simulink model "Mdl_Tacho"  (R2024b)
settings: Solver=FixedStepDiscrete  StartTime=0.0  StopTime=10.0  FixedStep=0.1  RelTol=1e-3  EnableMultiTasking=on
values from neighbouring files (symbols this model uses):
  EQUIPPED_FLAG = mpt.Parameter    [Mdl_Tacho_DD.m]
  HV_NE = mpt.Parameter    [Mdl_Tacho_DD.m]
  MCUID0025 = mpt.Parameter    [Mdl_Tacho_DD.m]
  MCUID0025_MAX = mpt.Parameter    [Mdl_Tacho_DD.m]
  MCUID0639 = mpt.Parameter    [Mdl_Tacho_DD.m]
  MCUID0640 = mpt.Parameter    [Mdl_Tacho_DD.m]
  Mdl_Tacho_cTaskPeriod = mpt.Parameter    [Mdl_Tacho_rte_types.m]
  N1 = mpt.Parameter    [Mdl_Tacho_DD.m]
  N2 = mpt.Parameter    [Mdl_Tacho_DD.m]
  NE1 = mpt.Parameter    [Mdl_Tacho_DD.m]
  NE_MET = mpt.Parameter    [Mdl_Tacho_DD.m]
  NE_MET_INVALID = mpt.Parameter    [Mdl_Tacho_DD.m]
  PTSYS_48V = mpt.Parameter    [Mdl_Tacho_DD.m]
  PTSYS_CONV = mpt.Parameter    [Mdl_Tacho_DD.m]
  PTSYS_DEFAULT = mpt.Parameter    [Mdl_Tacho_DD.m]
  PTSYS_HV = mpt.Parameter    [Mdl_Tacho_DD.m]
  PTSYS_MOTORHV = mpt.Parameter    [Mdl_Tacho_DD.m]
  PTSYS_PHV = mpt.Parameter    [Mdl_Tacho_DD.m]
  PTSYS_S_S = mpt.Parameter    [Mdl_Tacho_DD.m]
  REDZONE_MAX_VAL = mpt.Parameter    [Mdl_Tacho_DD.m]
  REDZONE_MIN_VAL = mpt.Parameter    [Mdl_Tacho_DD.m]
  RTE_E_MAX_AGE_EXCEEDED = mpt.Parameter    [Mdl_Tacho_rte_types.m]
  RTE_E_NEVER_RECEIVED = mpt.Parameter    [Mdl_Tacho_rte_types.m]
  RTE_E_OK = mpt.Parameter    [Mdl_Tacho_rte_types.m]
  RZ_INIT_VAL = mpt.Parameter    [Mdl_Tacho_DD.m]
  SPD_THRESHOLD = mpt.Parameter    [Mdl_Tacho_DD.m]
  TACHO_070D = mpt.Parameter    [Mdl_Tacho_DD.m]
  TACHO_COUNT_INIT = mpt.Parameter    [Mdl_Tacho_DD.m]
  TACHO_COUNT_INIT_U16 = mpt.Parameter    [Mdl_Tacho_DD.m]
  TACHO_COUNT_ONE = mpt.Parameter    [Mdl_Tacho_DD.m]
  TACHO_COUNT_TWO = mpt.Parameter    [Mdl_Tacho_DD.m]
  TACHO_DEBOUNCE_TIME = mpt.Parameter    [Mdl_Tacho_DD.m]
  TACHO_DISABLE = mpt.Parameter    [Mdl_Tacho_DD.m]
  TACHO_ENABLE = mpt.Parameter    [Mdl_Tacho_DD.m]
  TACHO_F = mpt.Parameter    [Mdl_Tacho_DD.m]
  TACHO_FSPORT = mpt.Parameter    [Mdl_Tacho_DD.m]
  TACHO_GR = mpt.Parameter    [Mdl_Tacho_DD.m]
  TACHO_GRMN = mpt.Parameter    [Mdl_Tacho_DD.m]
  TACHO_HYS_MAX = mpt.Parameter    [Mdl_Tacho_DD.m]
  TACHO_HYS_MIN = mpt.Parameter    [Mdl_Tacho_DD.m]
  TACHO_OFF = mpt.Parameter    [Mdl_Tacho_DD.m]
  TACHO_ON = mpt.Parameter    [Mdl_Tacho_DD.m]
  TACHO_RES_DIVIDER = mpt.Parameter    [Mdl_Tacho_DD.m]
  TACHO_RESOLUTION = mpt.Parameter    [Mdl_Tacho_DD.m]
  TACHO_REV_PEAK_TIMER_ELAPSED = mpt.Parameter    [Mdl_Tacho_DD.m]
  TACHO_RPM_THRESHOLD = mpt.Parameter    [Mdl_Tacho_DD.m]
  TACHO_TEN = mpt.Parameter    [Mdl_Tacho_DD.m]
  TACHO_THRESHOLD = mpt.Parameter    [Mdl_Tacho_DD.m]
  TACHO_VAL_ONE = mpt.Parameter    [Mdl_Tacho_DD.m]
  TACHO_VAL_ONE_U16 = mpt.Parameter    [Mdl_Tacho_DD.m]
  TACHO_VAL_TEN = mpt.Parameter    [Mdl_Tacho_DD.m]
  TACHO_VAL_THREE = mpt.Parameter    [Mdl_Tacho_DD.m]
  TACHO_VAL_TWENTY = mpt.Parameter    [Mdl_Tacho_DD.m]
  TACHO_VAL_ZERO = mpt.Parameter    [Mdl_Tacho_DD.m]
  TACHO_VAL_ZERO_U16 = mpt.Parameter    [Mdl_Tacho_DD.m]
  TACHO_VAL_ZERO_U32 = mpt.Parameter    [Mdl_Tacho_DD.m]
  VAL_ONE = mpt.Parameter    [Mdl_Tacho_DD.m]
  VAL_ZERO = mpt.Parameter    [Mdl_Tacho_DD.m]
undefined symbols (not defined in the file or in its folder): CLUSTER_ACTIVE, CLUSTER_INACTIVE, eEngineSpeedIn, eFUNC_NORTH_AMERICA, eJust_Received, eSIGNAL_MISSING, eSIGNAL_NEVER_RECEIVED, IgnOff, IgnOn, NE1_Recieve_Notify_Value, NE1_SignalVal, pJustRcvdStatus, RxCan_SignalClearJustRcvdStatus, RxCan_SignalGetJustRcvdStatus, RxCan_SignalInvalidProcessingControl, RxCan_SignalMissingProcessingControl, RxCan_SignalNRProcessingControl, SignalId, Status, tRxSignalId_type_instance, tRxSignalJustRcvdStatus_type_instance, tRxSignalStatus_type_instance
libraries: simulink x23
(part 2 of 3)

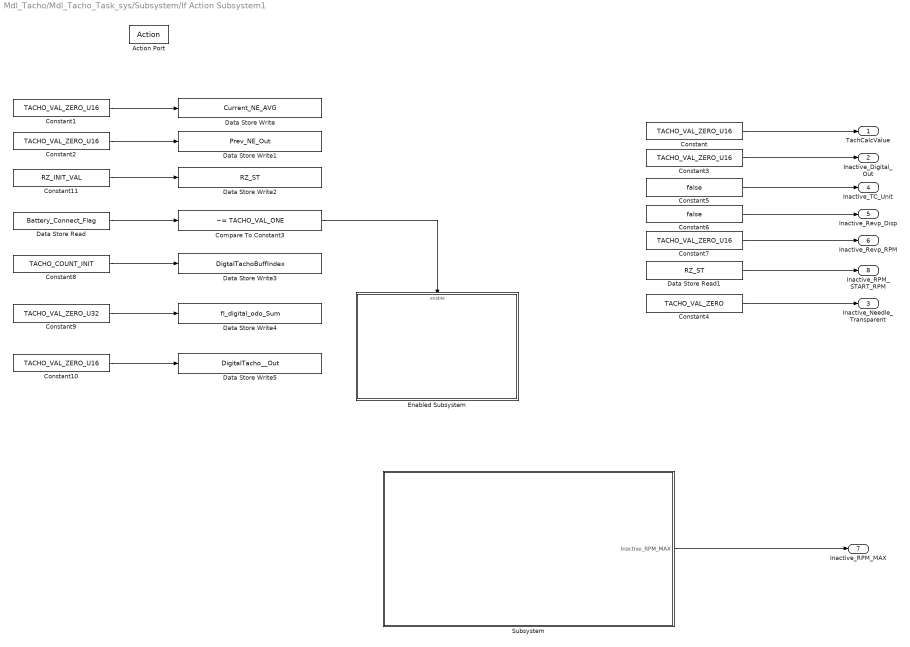
== system Mdl_Tacho/Mdl_Tacho_Task_sys/Subsystem/If Action Subsystem1 ==
  Action Port : ActionPort  ActionPortLabel=else
  Compare To Constant3 : simulink/Logic and Bit Operations/Compare To Constant  relop=~=  const=TACHO_VAL_ONE  OutDataTypeStr=boolean
  Constant{,1..3} (4 alike) : Constant  Value=TACHO_VAL_ZERO_U16  OutDataTypeStr=uint16  LockScale=on
  Constant10 : Constant  Value=TACHO_VAL_ZERO_U16  LockScale=on
  Constant11 : Constant  Value=RZ_INIT_VAL
  Constant4 : Constant  Value=TACHO_VAL_ZERO  LockScale=on
  Constant5 : Constant  Value=false  LockScale=on
  Constant6 : Constant  Value=false  LockScale=on
  Constant7 : Constant  Value=TACHO_VAL_ZERO_U16  LockScale=on
  Constant8 : Constant  Value=TACHO_COUNT_INIT
  Constant9 : Constant  Value=TACHO_VAL_ZERO_U32  LockScale=on
  Data Store Read : DataStoreRead  DataStoreName=Battery_Connect_Flag  IndexOptions=Index vector (dialog)  Indices=1  OutputSizes=1
  Data Store Read1 : DataStoreRead  DataStoreName=RZ_ST  IndexOptions=Index vector (dialog)  Indices=1  OutputSizes=1
  Data Store Write : DataStoreWrite  DataStoreName=Current_NE_AVG  IndexOptions=Index vector (dialog)  Indices=1  OutputSizes=1
  Data Store Write1 : DataStoreWrite  DataStoreName=Prev_NE_Out  IndexOptions=Index vector (dialog)  Indices=1  OutputSizes=1
  Data Store Write2 : DataStoreWrite  DataStoreName=RZ_ST  IndexOptions=Index vector (dialog)  Indices=1  OutputSizes=1
  Data Store Write3 : DataStoreWrite  DataStoreName=DigtalTachoBuffIndex  IndexOptions=Index vector (dialog)  Indices=1  OutputSizes=1
  Data Store Write4 : DataStoreWrite  DataStoreName=fl_digital_odo_Sum  IndexOptions=Index vector (dialog)  Indices=1  OutputSizes=1
  Data Store Write5 : DataStoreWrite  DataStoreName=DigitalTacho__Out  IndexOptions=Index vector (dialog)  Indices=1  OutputSizes=1
  Enabled Subsystem : Subsystem  Priority=0  TreatAsAtomicUnit=on
  Subsystem : Subsystem  Priority=1
  TachCalcValue : Outport  VectorParamsAs1DForOutWhenUnconnected=off
  Inactive_Digital_Out : Outport  Port=2  VectorParamsAs1DForOutWhenUnconnected=off
  Inactive_Needle_Transparent : Outport  Port=3  VectorParamsAs1DForOutWhenUnconnected=off
  Inactive_TC_Unit : Outport  Port=4  VectorParamsAs1DForOutWhenUnconnected=off
  Inactive_Revp_Disp : Outport  Port=5  VectorParamsAs1DForOutWhenUnconnected=off
  Inactive_Revp_RPM : Outport  Port=6  VectorParamsAs1DForOutWhenUnconnected=off
  Inactive_RPM_MAX : Outport  Port=7  VectorParamsAs1DForOutWhenUnconnected=off
  Inactive_RPM_START_RPM : Outport  Port=8  VectorParamsAs1DForOutWhenUnconnected=off
  wires:
  Constant/1 -> TachCalcValue/1
  Constant1/1 -> Data Store Write/1
  Constant2/1 -> Data Store Write1/1
  Constant3/1 -> Inactive_Digital_Out/1
  Constant4/1 -> Inactive_Needle_Transparent/1
  Constant5/1 -> Inactive_TC_Unit/1
  Constant6/1 -> Inactive_Revp_Disp/1
  Constant7/1 -> Inactive_Revp_RPM/1
  Data Store Read1/1 -> Inactive_RPM_START_RPM/1
  Constant11/1 -> Data Store Write2/1
  Data Store Read/1 -> Compare To Constant3/1
  Compare To Constant3/1 -> Enabled Subsystem/Enable
  Constant8/1 -> Data Store Write3/1
  Constant9/1 -> Data Store Write4/1
  Constant10/1 -> Data Store Write5/1
  Subsystem/1(Inactive_RPM_MAX) -> Inactive_RPM_MAX/1

== system Mdl_Tacho/Mdl_Tacho_Task_sys/Subsystem/NE1_Missing_Notify ==
  NE1_COMStatus : Inport
  NE1_Value : Inport  Port=2
  NE1_In_JR : Inport  Port=3
  Compare To Constant1 : simulink/Logic and Bit Operations/Compare To Constant  relop=~=  const=RTE_E_MAX_AGE_EXCEEDED  OutDataTypeStr=boolean
  If : If  IfExpression=u1 ~= 0
  If Action Subsystem : Subsystem  TreatAsAtomicUnit=on
  If Action Subsystem1 : Subsystem  TreatAsAtomicUnit=on
  Merge : Merge
  NE1_Status : Outport  VectorParamsAs1DForOutWhenUnconnected=off
  wires:
  NE1_COMStatus/1 -> Compare To Constant1/1
  Compare To Constant1/1 -> If/1
  If/1 -> If Action Subsystem/Action
  NE1_In_JR/1 -> If Action Subsystem/1(NE1_In_JR)
  If Action Subsystem/1(NE1_Status) -> Merge/1
  If Action Subsystem1/1(NE1_Status) -> Merge/2
  Merge/1 -> NE1_Status/1
  If/2 -> If Action Subsystem1/Action
  NE1_Value/1 -> If Action Subsystem/2(NE1_Value)

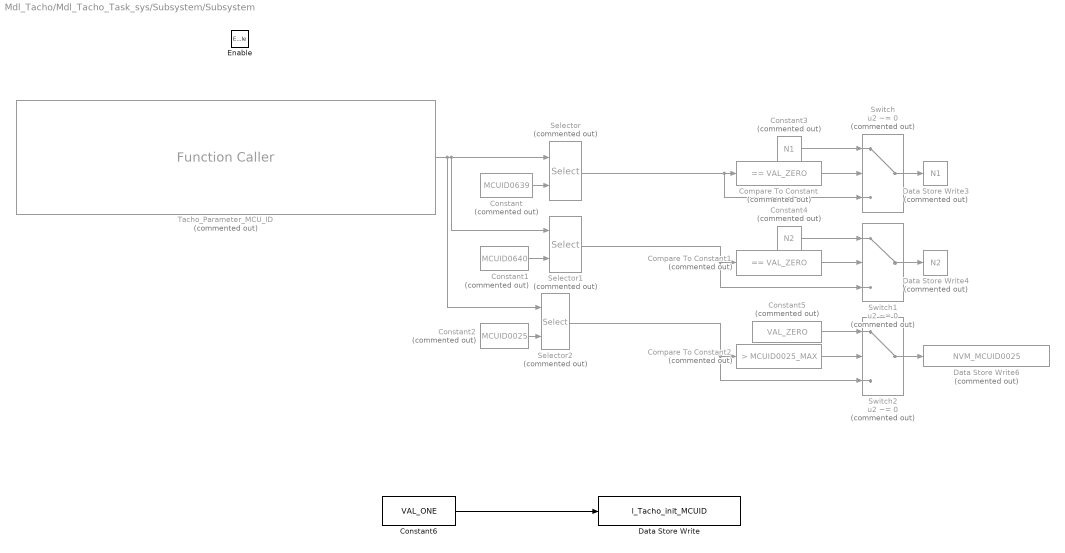
== system Mdl_Tacho/Mdl_Tacho_Task_sys/Subsystem/Subsystem ==
  Enable : EnablePort
  Compare To Constant : simulink/Logic and Bit Operations/Compare To Constant  Commented=on  relop===  const=VAL_ZERO  OutDataTypeStr=boolean
  Compare To Constant1 : simulink/Logic and Bit Operations/Compare To Constant  Commented=on  relop===  const=VAL_ZERO  OutDataTypeStr=boolean
  Compare To Constant2 : simulink/Logic and Bit Operations/Compare To Constant  Commented=on  relop=>  const=MCUID0025_MAX  OutDataTypeStr=boolean
  Constant : Constant  Commented=on  Value=MCUID0639
  Constant1 : Constant  Commented=on  Value=MCUID0640
  Constant2 : Constant  Commented=on  Value=MCUID0025
  Constant3 : Constant  Commented=on  Value=N1
  Constant4 : Constant  Commented=on  Value=N2
  Constant5 : Constant  Commented=on  Value=VAL_ZERO
  Constant6 : Constant  Value=VAL_ONE
  Data Store Write : DataStoreWrite  DataStoreName=l_Tacho_init_MCUID  IndexOptions=Index vector (dialog)  Indices=1  OutputSizes=1
  Data Store Write3 : DataStoreWrite  Commented=on  DataStoreName=N1  IndexOptions=Index vector (dialog)  Indices=1  OutputSizes=1
  Data Store Write4 : DataStoreWrite  Commented=on  DataStoreName=N2  IndexOptions=Index vector (dialog)  Indices=1  OutputSizes=1
  Data Store Write6 : DataStoreWrite  Commented=on  DataStoreName=NVM_MCUID0025  IndexOptions=Index vector (dialog)  Indices=1  OutputSizes=1
  Selector : Selector  Commented=on  IndexMode=Zero-based  InputPortWidth=6  IndexOptions=Index vector (port)  Indices=[1 3]  OutputSizes=1
  Selector1 : Selector  Commented=on  IndexMode=Zero-based  InputPortWidth=6  IndexOptions=Index vector (port)  Indices=[1 3]  OutputSizes=1
  Selector2 : Selector  Commented=on  IndexMode=Zero-based  InputPortWidth=6  IndexOptions=Index vector (port)  Indices=[1 3]  OutputSizes=1
  Switch : Switch  Commented=on  Criteria=u2 ~= 0  OutDataTypeStr=uint16  SaturateOnIntegerOverflow=off  InputSameDT=off
  Switch1 : Switch  Commented=on  Criteria=u2 ~= 0  OutDataTypeStr=uint16  SaturateOnIntegerOverflow=off  InputSameDT=off
  Switch2 : Switch  Commented=on  Criteria=u2 ~= 0  OutDataTypeStr=uint8  SaturateOnIntegerOverflow=off  InputSameDT=off
  Tacho_Parameter_MCU_ID : FunctionCaller  Commented=on  FunctionPrototype=pMCUCONST_Data = Tacho_Parameter_MCU_ID()  InputArgumentSpecifications=<Enter example>  OutputArgumentSpecifications=uint16(zeros(1,6))
  wires:
  Constant/1 -> Selector/2
  Constant1/1 -> Selector1/2
  Constant2/1 -> Selector2/2
  Selector/1 -> Switch/3, Compare To Constant/1
  Compare To Constant/1 -> Switch/2
  Compare To Constant1/1 -> Switch1/2
  Constant3/1 -> Switch/1
  Switch/1 -> Data Store Write3/1
  Constant4/1 -> Switch1/1
  Selector1/1 -> Switch1/3, Compare To Constant1/1
  Switch1/1 -> Data Store Write4/1
  Constant5/1 -> Switch2/1
  Compare To Constant2/1 -> Switch2/2
  Selector2/1 -> Switch2/3, Compare To Constant2/1
  Switch2/1 -> Data Store Write6/1
  Tacho_Parameter_MCU_ID/1 -> Selector1/1, Selector/1, Selector2/1
  Constant6/1 -> Data Store Write/1

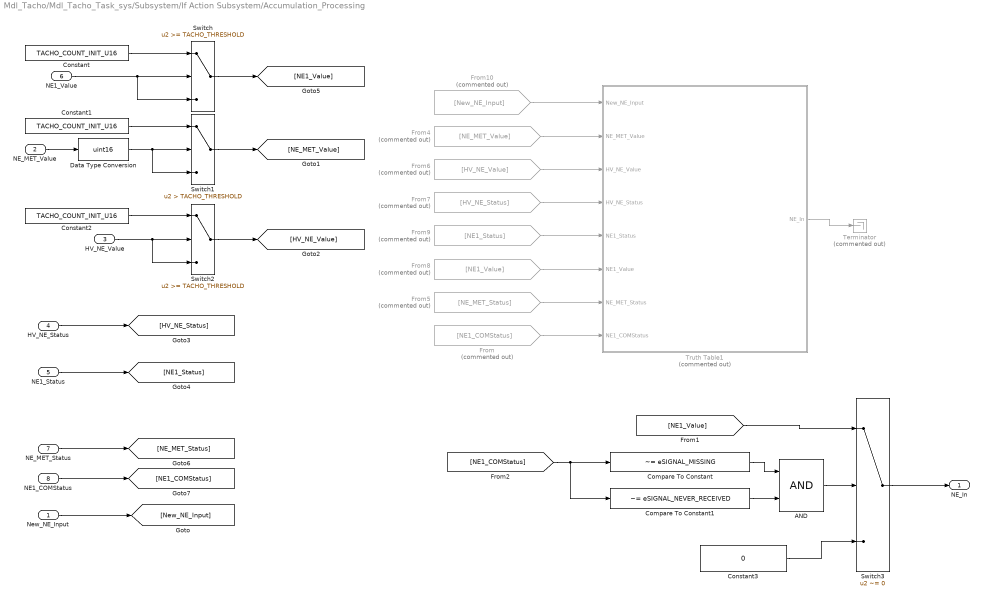
== system Mdl_Tacho/Mdl_Tacho_Task_sys/Subsystem/If Action Subsystem/Accumulation_Processing ==
  New_NE_Input : Inport
  NE_MET_Value : Inport  Port=2
  HV_NE_Value : Inport  Port=3
  HV_NE_Status : Inport  Port=4
  NE1_Status : Inport  Port=5
  NE1_Value : Inport  Port=6
  NE_MET_Status : Inport  Port=7
  NE1_COMStatus : Inport  Port=8
  AND : Logic  AllPortsSameDT=off  OutDataTypeStr=boolean
  Compare To Constant : simulink/Logic and Bit Operations/Compare To Constant  relop=~=  const=eSIGNAL_MISSING  OutDataTypeStr=boolean
  Compare To Constant1 : simulink/Logic and Bit Operations/Compare To Constant  relop=~=  const=eSIGNAL_NEVER_RECEIVED  OutDataTypeStr=boolean
  Constant : Constant  Value=TACHO_COUNT_INIT_U16
  Constant1 : Constant  Value=TACHO_COUNT_INIT_U16
  Constant2 : Constant  Value=TACHO_COUNT_INIT_U16
  Constant3 : Constant  Value=0
  Data Type Conversion : DataTypeConversion  OutDataTypeStr=uint16  SaturateOnIntegerOverflow=off  RndMeth=Floor
  From : From  Commented=on  GotoTag=NE1_COMStatus
  From10 : From  Commented=on  GotoTag=New_NE_Input
  From4 : From  Commented=on  GotoTag=NE_MET_Value
  From5 : From  Commented=on  GotoTag=NE_MET_Status
  From6 : From  Commented=on  GotoTag=HV_NE_Value
  From7 : From  Commented=on  GotoTag=HV_NE_Status
  From8 : From  Commented=on  GotoTag=NE1_Value
  From9 : From  Commented=on  GotoTag=NE1_Status
  Switch : Switch  Threshold=TACHO_THRESHOLD  OutDataTypeStr=uint16  SaturateOnIntegerOverflow=off  InputSameDT=off
  Switch1 : Switch  Criteria=u2 > Threshold  Threshold=TACHO_THRESHOLD  SaturateOnIntegerOverflow=off  InputSameDT=off
  Switch2 : Switch  Threshold=TACHO_THRESHOLD  SaturateOnIntegerOverflow=off  InputSameDT=off
  Switch3 : Switch  Criteria=u2 ~= 0  OutDataTypeStr=uint16  SaturateOnIntegerOverflow=off  InputSameDT=off
  Terminator : Terminator  Commented=on
  Truth Table1 : Truth Table  Commented=on  TreatAsAtomicUnit=on
  NE_In : Outport  VectorParamsAs1DForOutWhenUnconnected=off
  wires:
  From6/1 -> Truth Table1/3(HV_NE_Value)
  From9/1 -> Truth Table1/5(NE1_Status)
  From5/1 -> Truth Table1/7(NE_MET_Status)
  From7/1 -> Truth Table1/4(HV_NE_Status)
  From10/1 -> Truth Table1/1(New_NE_Input)
  From4/1 -> Truth Table1/2(NE_MET_Value)
  From8/1 -> Truth Table1/6(NE1_Value)
  HV_NE_Status/1 -> [HV_NE_Status]
  NE1_Status/1 -> [NE1_Status]
  NE_MET_Status/1 -> [NE_MET_Status]
  NE1_COMStatus/1 -> [NE1_COMStatus]
  From/1 -> Truth Table1/8(NE1_COMStatus)
  Constant/1 -> Switch/1
  Switch1/1 -> [NE_MET_Value]
  Constant1/1 -> Switch1/1
  NE_MET_Value/1 -> Data Type Conversion/1
  HV_NE_Value/1 -> Switch2/3, Switch2/2
  Constant2/1 -> Switch2/1
  Switch2/1 -> [HV_NE_Value]
  New_NE_Input/1 -> [New_NE_Input]
  Switch/1 -> [NE1_Value]
  NE1_Value/1 -> Switch/3, Switch/2
  [NE1_COMStatus] -> Compare To Constant1/1, Compare To Constant/1
  Compare To Constant/1 -> AND/1
  Compare To Constant1/1 -> AND/2
  Switch3/1 -> NE_In/1
  AND/1 -> Switch3/2
  [NE1_Value] -> Switch3/1
  Constant3/1 -> Switch3/3
  Truth Table1/1(NE_In) -> Terminator/1
  Data Type Conversion/1 -> Switch1/3, Switch1/2

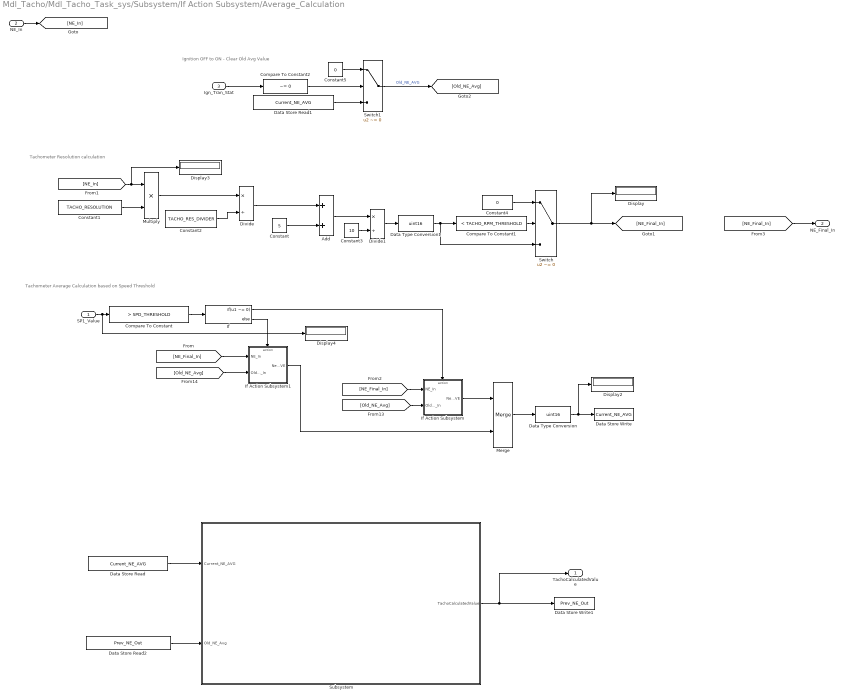
== system Mdl_Tacho/Mdl_Tacho_Task_sys/Subsystem/If Action Subsystem/Average_Calculation ==
  note: Tachometer Average Calculation based on Speed Threshold
  note: Tachometer Resolution calculation
  note: Ignition OFF to ON - Clear Old Avg Value
  SP1_Value : Inport
  NE_In : Inport  Port=2
  Ign_Tran_Stat : Inport  Port=3
  Add : Sum  OutDataTypeStr=uint32  RndMeth=Simplest
  Compare To Constant : simulink/Logic and Bit Operations/Compare To Constant  relop=>  const=SPD_THRESHOLD  OutDataTypeStr=boolean
  Compare To Constant1 : simulink/Logic and Bit Operations/Compare To Constant  relop=<  const=TACHO_RPM_THRESHOLD  OutDataTypeStr=boolean
  Compare To Constant2 : simulink/Logic and Bit Operations/Compare To Constant  relop=~=  const=0  OutDataTypeStr=boolean
  Constant : Constant  Value=5  OutDataTypeStr=uint16  LockScale=on
  Constant1 : Constant  Value=TACHO_RESOLUTION  OutDataTypeStr=uint32  LockScale=on
  Constant2 : Constant  Value=TACHO_RES_DIVIDER  OutDataTypeStr=uint32  LockScale=on
  Constant3 : Constant  Value=10  OutDataTypeStr=uint16  LockScale=on
  Constant4 : Constant  Value=0  OutDataTypeStr=uint16  LockScale=on
  Constant5 : Constant  Value=0  OutDataTypeStr=uint16
  Data Store Read : DataStoreRead  DataStoreName=Current_NE_AVG  IndexOptions=Index vector (dialog)  Indices=1  OutputSizes=1
  Data Store Read1 : DataStoreRead  DataStoreName=Current_NE_AVG  IndexOptions=Index vector (dialog)  Indices=1  OutputSizes=1
  Data Store Read2 : DataStoreRead  DataStoreName=Prev_NE_Out  IndexOptions=Index vector (dialog)  Indices=1  OutputSizes=1
  Data Store Write : DataStoreWrite  DataStoreName=Current_NE_AVG  IndexOptions=Index vector (dialog)  Indices=1  OutputSizes=1
  Data Store Write1 : DataStoreWrite  DataStoreName=Prev_NE_Out  IndexOptions=Index vector (dialog)  Indices=1  OutputSizes=1
  Data Type Conversion : DataTypeConversion  OutDataTypeStr=uint16  RndMeth=Simplest  SaturateOnIntegerOverflow=off
  Data Type Conversion1 : DataTypeConversion  OutDataTypeStr=uint16  RndMeth=Simplest  SaturateOnIntegerOverflow=off
  Display{,2..4} (4 alike) : Display
  Divide : Product  Inputs=*/  OutDataTypeStr=uint32  RndMeth=Simplest
  Divide1 : Product  Inputs=*/  OutDataTypeStr=uint32  RndMeth=Simplest
  If : If  Priority=3  IfExpression=u1 ~= 0
  If Action Subsystem : Subsystem  TreatAsAtomicUnit=on
  If Action Subsystem1 : Subsystem  TreatAsAtomicUnit=on
  Merge : Merge
  Multiply : Product  OutDataTypeStr=uint32  RndMeth=Simplest  LockScale=on
  Subsystem : Subsystem  Priority=4  TreatAsAtomicUnit=on  RTWFcnName=Mdl_Tacho_Hysteris_Process_Output
      settings: RTWSystemCode=Nonreusable function  RTWFcnNameOpts=User specified
  Switch : Switch  Priority=2  Criteria=u2 ~= 0  OutDataTypeStr=uint16  RndMeth=Simplest  SaturateOnIntegerOverflow=off  InputSameDT=off
  Switch1 : Switch  Priority=1  Criteria=u2 ~= 0  OutDataTypeStr=uint16  RndMeth=Simplest  SaturateOnIntegerOverflow=off  InputSameDT=off
  TachoCalculatedValue : Outport  VectorParamsAs1DForOutWhenUnconnected=off
  NE_Final_In : Outport  Port=2  VectorParamsAs1DForOutWhenUnconnected=off
  wires:
  If Action Subsystem/1(New NE_AVE) -> Merge/1
  [NE_Final_In] -> If Action Subsystem/1(NE_In)
  If/1 -> If Action Subsystem/Action
  [Old_NE_Avg] -> If Action Subsystem/2(Old_NE_In)
  If/2 -> If Action Subsystem1/Action
  Merge/1 -> Data Type Conversion/1
  Compare To Constant/1 -> If/1
  [Old_NE_Avg] -> If Action Subsystem1/2(Old_NE_In)
  If Action Subsystem1/1(New NE_AVE) -> Merge/2
  NE_In/1 -> [NE_In]
  Constant1/1 -> Multiply/2
  [NE_Final_In] -> If Action Subsystem1/1(NE_In)
  Multiply/1 -> Divide/1
  Constant2/1 -> Divide/2
  Divide/1 -> Add/1
  Constant/1 -> Add/2
  Add/1 -> Divide1/1
  Constant3/1 -> Divide1/2
  Divide1/1 -> Data Type Conversion1/1
  Compare To Constant1/1 -> Switch/2
  Constant4/1 -> Switch/1
  Switch/1 -> Display/1, [NE_Final_In]
  Ign_Tran_Stat/1 -> Compare To Constant2/1
  Compare To Constant2/1 -> Switch1/2
  Switch1/1 -> [Old_NE_Avg]  "Old_NE_AVG"
  Constant5/1 -> Switch1/1
  Data Store Read1/1 -> Switch1/3
  Data Type Conversion1/1 -> Compare To Constant1/1, Switch/3
  SP1_Value/1 -> Display4/1, Compare To Constant/1
  Data Store Read/1 -> Subsystem/1(Current_NE_AVG)
  Data Store Read2/1 -> Subsystem/2(Old_NE_Avg)
  Subsystem/1(TachoCalculatedValue) -> Data Store Write1/1, TachoCalculatedValue/1
  Data Type Conversion/1 -> Display2/1, Data Store Write/1
  [NE_In] -> Display3/1, Multiply/1
  [NE_Final_In] -> NE_Final_In/1

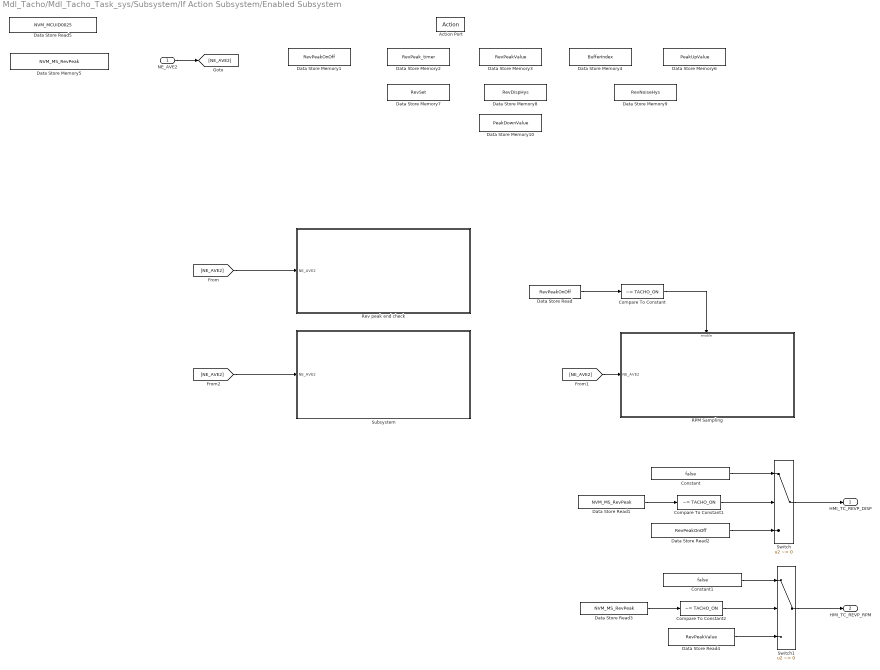
== system Mdl_Tacho/Mdl_Tacho_Task_sys/Subsystem/If Action Subsystem/Enabled Subsystem ==
  NE_AVE2 : Inport
  Action Port : ActionPort
  Compare To Constant : simulink/Logic and Bit Operations/Compare To Constant  relop=~=  const=TACHO_ON  OutDataTypeStr=boolean
  Compare To Constant1 : simulink/Logic and Bit Operations/Compare To Constant  relop=~=  const=TACHO_ON  OutDataTypeStr=boolean
  Compare To Constant2 : simulink/Logic and Bit Operations/Compare To Constant  relop=~=  const=TACHO_ON  OutDataTypeStr=boolean
  Constant : Constant  Value=false
  Constant1 : Constant  Value=false
  Data Store Memory1 : DataStoreMemory  DataStoreName=RevPeakOnOff  ReadBeforeWriteMsg=warning  WriteAfterWriteMsg=warning  WriteAfterReadMsg=warning  InitialValue=false  ShowAdditionalParam=off  OutDataTypeStr=boolean
  Data Store Memory10 : DataStoreMemory  DataStoreName=PeakDownValue  ReadBeforeWriteMsg=warning  WriteAfterWriteMsg=warning  WriteAfterReadMsg=warning  InitialValue=TACHO_VAL_ZERO_U16  ShowAdditionalParam=off  OutDataTypeStr=uint16
  Data Store Memory2 : DataStoreMemory  DataStoreName=RevPeak_timer  ReadBeforeWriteMsg=warning  WriteAfterWriteMsg=warning  WriteAfterReadMsg=warning  InitialValue=TACHO_VAL_ZERO_U16  ShowAdditionalParam=off  OutDataTypeStr=uint16
  Data Store Memory3 : DataStoreMemory  DataStoreName=RevPeakValue  ReadBeforeWriteMsg=warning  WriteAfterWriteMsg=warning  WriteAfterReadMsg=warning  InitialValue=TACHO_VAL_ZERO_U16  ShowAdditionalParam=off  OutDataTypeStr=uint16
  Data Store Memory4 : DataStoreMemory  DataStoreName=BufferIndex  ReadBeforeWriteMsg=warning  WriteAfterWriteMsg=warning  WriteAfterReadMsg=warning  InitialValue=TACHO_VAL_ZERO  ShowAdditionalParam=off  OutDataTypeStr=uint8
  Data Store Memory5 : DataStoreMemory  DataStoreName=NVM_MS_RevPeak  ReadBeforeWriteMsg=warning  WriteAfterWriteMsg=warning  WriteAfterReadMsg=warning  InitialValue=TACHO_VAL_ZERO  ShowAdditionalParam=off
  Data Store Memory6 : DataStoreMemory  DataStoreName=PeakUpValue  ReadBeforeWriteMsg=warning  WriteAfterWriteMsg=warning  WriteAfterReadMsg=warning  InitialValue=TACHO_VAL_ZERO_U16  ShowAdditionalParam=off  OutDataTypeStr=uint16
  Data Store Memory7 : DataStoreMemory  DataStoreName=RevSet  ReadBeforeWriteMsg=warning  WriteAfterWriteMsg=warning  WriteAfterReadMsg=warning  InitialValue=TACHO_VAL_ZERO_U16  ShowAdditionalParam=off  OutDataTypeStr=uint16
  Data Store Memory8 : DataStoreMemory  DataStoreName=RevDispHys  ReadBeforeWriteMsg=warning  WriteAfterWriteMsg=warning  WriteAfterReadMsg=warning  InitialValue=TACHO_VAL_ZERO_U16  ShowAdditionalParam=off  OutDataTypeStr=uint16
  Data Store Memory9 : DataStoreMemory  DataStoreName=RevNoiseHys  ReadBeforeWriteMsg=warning  WriteAfterWriteMsg=warning  WriteAfterReadMsg=warning  InitialValue=TACHO_VAL_ZERO_U16  ShowAdditionalParam=off  OutDataTypeStr=uint16
  Data Store Read : DataStoreRead  DataStoreName=RevPeakOnOff  IndexOptions=Index vector (dialog)  Indices=1  OutputSizes=1
  Data Store Read1 : DataStoreRead  DataStoreName=NVM_MS_RevPeak  IndexOptions=Index vector (dialog)  Indices=1  OutputSizes=1
  Data Store Read2 : DataStoreRead  DataStoreName=RevPeakOnOff  IndexOptions=Index vector (dialog)  Indices=1  OutputSizes=1
  Data Store Read3 : DataStoreRead  DataStoreName=NVM_MS_RevPeak  IndexOptions=Index vector (dialog)  Indices=1  OutputSizes=1
  Data Store Read4 : DataStoreRead  DataStoreName=RevPeakValue  IndexOptions=Index vector (dialog)  Indices=1  OutputSizes=1
  Data Store Read5 : DataStoreRead  DataStoreName=NVM_MCUID0025  IndexOptions=Index vector (dialog)  Indices=1  OutputSizes=1
  RPM Sampling : Subsystem  TreatAsAtomicUnit=on
  Rev peak end check : Subsystem
  Subsystem : Subsystem
  Switch : Switch  Criteria=u2 ~= 0  SaturateOnIntegerOverflow=off  InputSameDT=off
  Switch1 : Switch  Criteria=u2 ~= 0  SaturateOnIntegerOverflow=off  InputSameDT=off
  HMI_TC_REVP_DISP : Outport  VectorParamsAs1DForOutWhenUnconnected=off
  HMI_TC_REVP_RPM : Outport  Port=2  VectorParamsAs1DForOutWhenUnconnected=off
  wires:
  NE_AVE2/1 -> [NE_AVE2]
  [NE_AVE2] -> Rev peak end check/1(NE_AVE2)
  Data Store Read/1 -> Compare To Constant/1
  Compare To Constant/1 -> RPM Sampling/Enable
  [NE_AVE2] -> RPM Sampling/1(NE_AVE2)
  [NE_AVE2] -> Subsystem/1(NE_AVE2)
  Data Store Read1/1 -> Compare To Constant1/1
  Compare To Constant1/1 -> Switch/2
  Constant/1 -> Switch/1
  Data Store Read2/1 -> Switch/3
  Switch/1 -> HMI_TC_REVP_DISP/1
  Switch1/1 -> HMI_TC_REVP_RPM/1
  Data Store Read3/1 -> Compare To Constant2/1
  Compare To Constant2/1 -> Switch1/2
  Constant1/1 -> Switch1/1
  Data Store Read4/1 -> Switch1/3

== system Mdl_Tacho/Mdl_Tacho_Task_sys/Subsystem/If Action Subsystem/Enabled Subsystem1 ==
  Action Port : ActionPort
  Constant : Constant  Value=false
  Constant1 : Constant  Value=TACHO_VAL_ZERO_U16
  HMI_TC_REVP_DISP : Outport  VectorParamsAs1DForOutWhenUnconnected=off
  HMI_TC_REVP_RPM : Outport  Port=2  VectorParamsAs1DForOutWhenUnconnected=off
  wires:
  Constant/1 -> HMI_TC_REVP_DISP/1
  Constant1/1 -> HMI_TC_REVP_RPM/1

== system Mdl_Tacho/Mdl_Tacho_Task_sys/Subsystem/If Action Subsystem/Input_Determination ==
  NE_MET_Ex : Inport
  HV_NE_Ex : Inport  Port=2
  Truth Table : Truth Table  TreatAsAtomicUnit=on
  New_NE_Input : Outport  VectorParamsAs1DForOutWhenUnconnected=off
  wires:
  [HV_NE_Ex] -> Truth Table/2(HV_NE_Ex)
  [NE_MET_Ex] -> Truth Table/1(NE_MET_Ex)
  Truth Table/1(New_NE_Input) -> New_NE_Input/1
  NE_MET_Ex/1 -> [NE_MET_Ex]
  HV_NE_Ex/1 -> [HV_NE_Ex]

== system Mdl_Tacho/Mdl_Tacho_Task_sys/Subsystem/If Action Subsystem/Subsystem ==
  NE_In : Inport
  Display : Display
  Subsystem : Subsystem
  Subsystem1 : Subsystem
  Digital_Tacho_Out : Outport  VectorParamsAs1DForOutWhenUnconnected=off
  wires:
  NE_In/1 -> Subsystem/1(NE_In)
  Subsystem/1(NE_IN_ForDigitalTacho) -> Subsystem1/1(NE_IN_ForDigitalTacho_In)
  Subsystem1/1(NE_IN_ForDigitalTacho_Out) -> Display/1, Digital_Tacho_Out/1

== system Mdl_Tacho/Mdl_Tacho_Task_sys/Subsystem/If Action Subsystem1/Enabled Subsystem ==
  Enable : EnablePort
  Constant : Constant  Value=TACHO_VAL_ONE
  Constant10 : Constant  Value=RZ_INIT_VAL
  Data Store Write : DataStoreWrite  DataStoreName=Battery_Connect_Flag  IndexOptions=Index vector (dialog)  Indices=1  OutputSizes=1
  Data Store Write3 : DataStoreWrite  DataStoreName=BURAM_RZ_MAX  IndexOptions=Index vector (dialog)  Indices=1  OutputSizes=1
  wires:
  Constant/1 -> Data Store Write/1
  Constant10/1 -> Data Store Write3/1

== system Mdl_Tacho/Mdl_Tacho_Task_sys/Subsystem/If Action Subsystem1/Subsystem ==
  Add : Sum  AccumDataTypeStr=uint8
  Add1 : Sum  AccumDataTypeStr=uint8
  Constant{12..16} (5 alike) : Constant  Value=TACHO_TEN
  Data Store Read2 : DataStoreRead  DataStoreName=BURAM_RZ_MAX  IndexOptions=Index vector (dialog)  Indices=1  OutputSizes=1
  Data Store Read3 : DataStoreRead  DataStoreName=BURAM_RZ_MAX  IndexOptions=Index vector (dialog)  Indices=1  OutputSizes=1
  Data Store Read5 : DataStoreRead  DataStoreName=BURAM_RZ_MAX  IndexOptions=Index vector (dialog)  Indices=1  OutputSizes=1
  Divide : Product  Inputs=*/
  Mod : Math  Operator=mod  SignedPower=on
  Multiply : Product  OutDataTypeStr=uint8
  Switch1 : Switch  Criteria=u2 ~= 0  OutDataTypeStr=uint8  SaturateOnIntegerOverflow=off  InputSameDT=off
  Inactive_RPM_MAX : Outport  VectorParamsAs1DForOutWhenUnconnected=off
  wires:
  Constant13/1 -> Divide/2
  Constant15/1 -> Multiply/2
  Constant14/1 -> Add/2
  Divide/1 -> Multiply/1
  Constant12/1 -> Mod/2
  Mod/1 -> Switch1/2
  Switch1/1 -> Add1/1
  Data Store Read2/1 -> Mod/1
  Data Store Read5/1 -> Divide/1
  Constant16/1 -> Add1/2
  Add/1 -> Switch1/1
  Multiply/1 -> Add/1
  Data Store Read3/1 -> Switch1/3
  Add1/1 -> Inactive_RPM_MAX/1

== system Mdl_Tacho/Mdl_Tacho_Task_sys/Subsystem/NE1_Missing_Notify/If Action Subsystem ==
  NE1_In_JR : Inport
  NE1_Value : Inport  Port=2
  Action Port : ActionPort  ActionPortLabel=if(u1 ~= 0)
  Compare To Constant : simulink/Logic and Bit Operations/Compare To Constant  relop===  const=eJust_Received  OutDataTypeStr=boolean
  Constant : Constant  Value=TACHO_DEBOUNCE_TIME
  Constant1 : Constant  Value=RTE_E_OK
  Constant2 : Constant  Value=RTE_E_MAX_AGE_EXCEEDED
  Constant3 : Constant  Value=Mdl_Tacho_cTaskPeriod
  Debounce timer Subsystem : Subsystem  Description=|
      | Input 1 : Deboune Count
      | Input 2 : Reset Timer Status
      | Output : Timer Debounce Status
  Divide : Product  Inputs=*/  OutDataTypeStr=uint8  RndMeth=Simplest
  Enabled Subsystem : Subsystem  Commented=on  TreatAsAtomicUnit=on
  Switch : Switch  Criteria=u2 ~= 0  SaturateOnIntegerOverflow=off  InputSameDT=off
  NE1_Status : Outport  VectorParamsAs1DForOutWhenUnconnected=off
  wires:
  Debounce timer Subsystem/1(TimerDebouncestatus) -> Switch/2
  Constant/1 -> Divide/1
  Compare To Constant/1 -> [JustReceivedStatus], Debounce timer Subsystem/2("ResetTimerStatus ")
  Divide/1 -> Debounce timer Subsystem/1(Debounce_Count)
  Constant2/1 -> Switch/1
  NE1_In_JR/1 -> Compare To Constant/1
  Constant1/1 -> Switch/3
  Constant3/1 -> Divide/2
  Switch/1 -> NE1_Status/1
  [JustReceivedStatus] -> Enabled Subsystem/Enable
  NE1_Value/1 -> Enabled Subsystem/1(NE1_Value)

== system Mdl_Tacho/Mdl_Tacho_Task_sys/Subsystem/NE1_Missing_Notify/If Action Subsystem1 ==
  Action Port : ActionPort  ActionPortLabel=else
  Constant : Constant  Value=RTE_E_MAX_AGE_EXCEEDED
  NE1_Status : Outport  VectorParamsAs1DForOutWhenUnconnected=off
  wires:
  Constant/1 -> NE1_Status/1

== system Mdl_Tacho/Mdl_Tacho_Task_sys/Subsystem/If Action Subsystem/Average_Calculation/If Action Subsystem ==
  NE_In : Inport
  Old_NE_In : Inport  Port=2
  Action Port : ActionPort  ActionPortLabel=if(u1 ~= 0)
  Add : Sum  OutDataTypeStr=uint32  AccumDataTypeStr=uint32  RndMeth=Simplest
  Constant1 : Constant  OutDataTypeStr=uint16  LockScale=on
  Data Store Read : DataStoreRead  DataStoreName=N1  IndexOptions=Index vector (dialog)  Indices=1  OutputSizes=1
  Data Store Read1 : DataStoreRead  DataStoreName=N1  IndexOptions=Index vector (dialog)  Indices=1  OutputSizes=1
  Data Type Conversion : DataTypeConversion  OutDataTypeStr=uint32  RndMeth=Simplest  SaturateOnIntegerOverflow=off
  Display : Display
  Divide : Product  Inputs=*/  OutDataTypeStr=uint16  RndMeth=Simplest
  Multiply : Product  OutDataTypeStr=uint32  RndMeth=Simplest
  Subtract : Sum  Inputs=+-  OutDataTypeStr=uint16  AccumDataTypeStr=uint16  RndMeth=Simplest
  New NE_AVE : Outport  VectorParamsAs1DForOutWhenUnconnected=off
  wires:
  Old_NE_In/1 -> Multiply/2
  Data Store Read/1 -> Subtract/1
  Constant1/1 -> Subtract/2
  NE_In/1 -> Data Type Conversion/1
  Multiply/1 -> Add/2
  Add/1 -> Divide/1
  Data Store Read1/1 -> Divide/2
  Divide/1 -> Display/1, New NE_AVE/1
  Subtract/1 -> Multiply/1
  Data Type Conversion/1 -> Add/1

== system Mdl_Tacho/Mdl_Tacho_Task_sys/Subsystem/If Action Subsystem/Average_Calculation/If Action Subsystem1 ==
  NE_In : Inport
  Old_NE_In : Inport  Port=2
  Action Port : ActionPort  ActionPortLabel=else
  Add : Sum  OutDataTypeStr=uint32  AccumDataTypeStr=uint32  RndMeth=Simplest
  Constant1 : Constant  OutDataTypeStr=uint16  LockScale=on
  Data Store Read : DataStoreRead  DataStoreName=N2  IndexOptions=Index vector (dialog)  Indices=1  OutputSizes=1
  Data Store Read1 : DataStoreRead  DataStoreName=N2  IndexOptions=Index vector (dialog)  Indices=1  OutputSizes=1
  Data Type Conversion : DataTypeConversion  OutDataTypeStr=uint32  RndMeth=Simplest  SaturateOnIntegerOverflow=off
  Display : Display
  Divide : Product  Inputs=*/  OutDataTypeStr=uint16  RndMeth=Simplest
  Multiply : Product  OutDataTypeStr=uint32  RndMeth=Simplest
  Subtract : Sum  Inputs=+-  OutDataTypeStr=uint16  AccumDataTypeStr=uint16  RndMeth=Simplest
  New NE_AVE : Outport  VectorParamsAs1DForOutWhenUnconnected=off
  wires:
  Subtract/1 -> Multiply/1
  NE_In/1 -> Data Type Conversion/1
  Data Store Read1/1 -> Divide/2
  Add/1 -> Divide/1
  Data Store Read/1 -> Subtract/1
  Constant1/1 -> Subtract/2
  Old_NE_In/1 -> Multiply/2
  Multiply/1 -> Add/2
  Divide/1 -> Display/1, New NE_AVE/1
  Data Type Conversion/1 -> Add/1

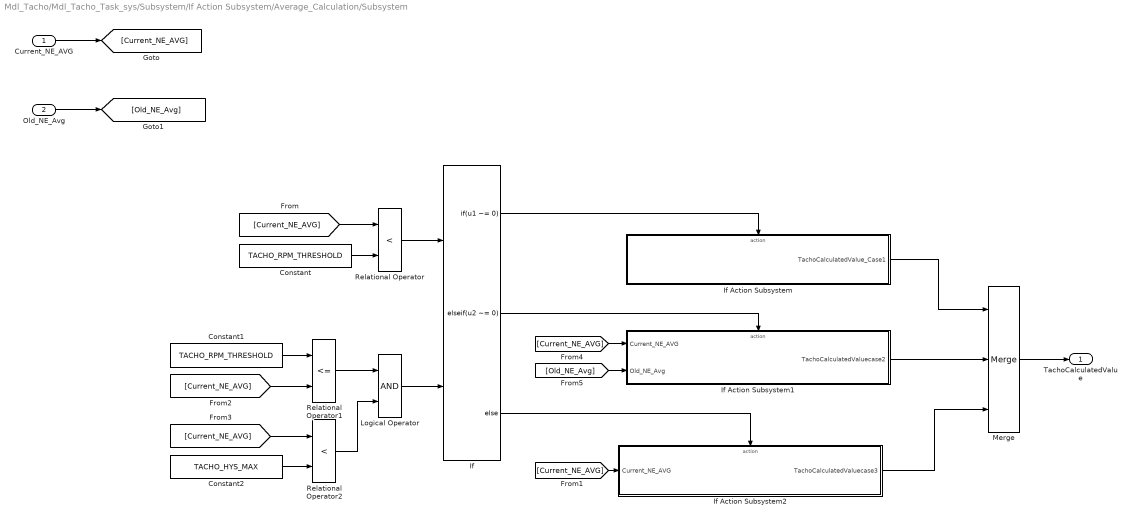
== system Mdl_Tacho/Mdl_Tacho_Task_sys/Subsystem/If Action Subsystem/Average_Calculation/Subsystem ==
  Current_NE_AVG : Inport
  Old_NE_Avg : Inport  Port=2
  Constant : Constant  Value=TACHO_RPM_THRESHOLD
  Constant1 : Constant  Value=TACHO_RPM_THRESHOLD
  Constant2 : Constant  Value=TACHO_HYS_MAX
  If : If  NumInputs=2  IfExpression=u1 ~= 0  ElseIfExpressions=u2 ~= 0
  If Action Subsystem : Subsystem  TreatAsAtomicUnit=on
  If Action Subsystem1 : Subsystem  TreatAsAtomicUnit=on
  If Action Subsystem2 : Subsystem  TreatAsAtomicUnit=on
  Logical Operator : Logic  AllPortsSameDT=off  OutDataTypeStr=boolean
  Merge : Merge  Inputs=3
  Relational Operator : RelationalOperator  Operator=<  OutDataTypeStr=boolean  RndMeth=Simplest  InputSameDT=off
  Relational Operator1 : RelationalOperator  Operator=<=  OutDataTypeStr=boolean  RndMeth=Simplest  InputSameDT=off
  Relational Operator2 : RelationalOperator  Operator=<  OutDataTypeStr=boolean  RndMeth=Simplest  InputSameDT=off
  TachoCalculatedValue : Outport  VectorParamsAs1DForOutWhenUnconnected=off
  wires:
  Current_NE_AVG/1 -> [Current_NE_AVG]
  Old_NE_Avg/1 -> [Old_NE_Avg]
  [Current_NE_AVG] -> Relational Operator/1
  Constant/1 -> Relational Operator/2
  Constant1/1 -> Relational Operator1/1
  [Current_NE_AVG] -> Relational Operator1/2
  Relational Operator1/1 -> Logical Operator/1
  [Current_NE_AVG] -> Relational Operator2/1
  Constant2/1 -> Relational Operator2/2
  Relational Operator2/1 -> Logical Operator/2
  Relational Operator/1 -> If/1
  Logical Operator/1 -> If/2
  If/1 -> If Action Subsystem/Action
  If/2 -> If Action Subsystem1/Action
  [Current_NE_AVG] -> If Action Subsystem1/1(Current_NE_AVG)
  [Old_NE_Avg] -> If Action Subsystem1/2(Old_NE_Avg)
  If/3 -> If Action Subsystem2/Action
  [Current_NE_AVG] -> If Action Subsystem2/1(Current_NE_AVG)
  If Action Subsystem/1("TachoCalculatedValue_Case1 ") -> Merge/1
  If Action Subsystem1/1(TachoCalculatedValuecase2) -> Merge/2
  If Action Subsystem2/1(TachoCalculatedValuecase3) -> Merge/3
  Merge/1 -> TachoCalculatedValue/1

== system Mdl_Tacho/Mdl_Tacho_Task_sys/Subsystem/If Action Subsystem/Enabled Subsystem/RPM Sampling ==
  NE_AVE2 : Inport
  Enable : EnablePort
  Data Store Read2 : DataStoreRead  DataStoreName=RevSet  IndexOptions=Index vector (dialog)  Indices=1  OutputSizes=1
  Data Store Read3 : DataStoreRead  DataStoreName=RevNoiseHys  IndexOptions=Index vector (dialog)  Indices=1  OutputSizes=1
  Data Store Read4 : DataStoreRead  DataStoreName=RevDispHys  IndexOptions=Index vector (dialog)  Indices=1  OutputSizes=1
  If : If  NumInputs=6  IfExpression=(u1 >= u4)&(u2 >= u6)&(u3 >= u5)  ShowElse=off
  If Action Subsystem : Subsystem  TreatAsAtomicUnit=on
  Subsystem : Subsystem
  Subsystem1 : Subsystem
  Subsystem2 : Subsystem
  Timer : Subsystem
  wires:
  NE_AVE2/1 -> [NE_AVE2]
  [NE_AVE2] -> Subsystem/1(NE_AVE2)
  [NE_AVE2] -> If/1
  Subsystem1/1(b) -> If/3
  [NE_AVE2] -> Subsystem2/1(NE_AVE2)
  Subsystem2/1(a) -> If/2
  Data Store Read3/1 -> If/5
  Data Store Read2/1 -> If/4
  Data Store Read4/1 -> If/6
  If/1 -> If Action Subsystem/Action
  [NE_AVE2] -> If Action Subsystem/1(NE_AVE2)

== system Mdl_Tacho/Mdl_Tacho_Task_sys/Subsystem/If Action Subsystem/Enabled Subsystem/Rev peak end check ==
  NE_AVE2 : Inport
  Add : Sum
  Constant1 : Constant  Value=TACHO_VAL_ONE
  Data Store Read : DataStoreRead  DataStoreName=RevPeak_timer  IndexOptions=Index vector (dialog)  Indices=1  OutputSizes=1
  Rev peak end check : Truth Table  TreatAsAtomicUnit=on
  wires:
  NE_AVE2/1 -> Rev peak end check/1(NE_AVE2)
  Data Store Read/1 -> Add/2
  Constant1/1 -> Add/1
  Add/1 -> Rev peak end check/2(RevPeakTimer_Plus_One)

== system Mdl_Tacho/Mdl_Tacho_Task_sys/Subsystem/If Action Subsystem/Enabled Subsystem/Subsystem ==
  NE_AVE2 : Inport  OutDataTypeStr=uint16
  Constant : Constant  Value=TACHO_VAL_ONE
  Data Store Read : DataStoreRead  DataStoreName=RevPeakOnOff  IndexOptions=Index vector (dialog)  Indices=1  OutputSizes=1
  Data Store Read1 : DataStoreRead  DataStoreName=PeakDownValue  IndexOptions=Index vector (dialog)  Indices=1  OutputSizes=1
  Data Type Conversion : DataTypeConversion  OutDataTypeStr=uint16  SaturateOnIntegerOverflow=off  RndMeth=Floor
  Data Type Conversion1 : DataTypeConversion  OutDataTypeStr=uint16  SaturateOnIntegerOverflow=off  RndMeth=Floor
  If : If  NumInputs=4  IfExpression=u3 > u1  ElseIfExpressions=(u2 == u4) & (u3 <= u1)  ShowElse=off
  If Action Subsystem : Subsystem  TreatAsAtomicUnit=on
  If Action Subsystem1 : Subsystem  TreatAsAtomicUnit=on
  wires:
  Data Store Read1/1 -> If/3
  Data Store Read/1 -> Data Type Conversion/1
  Constant/1 -> Data Type Conversion1/1
  If/1 -> If Action Subsystem/Action
  If/2 -> If Action Subsystem1/Action
  NE_AVE2/1 -> [NE_AVE2]
  [NE_AVE2] -> If/1
  [NE_AVE2] -> If Action Subsystem/1(NE_AVE2)
  Data Type Conversion/1 -> If/2
  Data Type Conversion1/1 -> If/4

== system Mdl_Tacho/Mdl_Tacho_Task_sys/Subsystem/If Action Subsystem/Subsystem/Subsystem ==
  NE_In : Inport
  Assignment : Assignment  IndexMode=Zero-based  OutputInitialize=Specify size for each dimension in table  DiagnosticForDimensions=Warning  IndexOptions=Index vector (port)  Indices=1  OutputSizes=3
  Data Store Read : DataStoreRead  DataStoreName=DigtalTachoBuffIndex  IndexOptions=Index vector (dialog)  Indices=1  OutputSizes=1
  NE_IN_ForDigitalTacho : Outport  VectorParamsAs1DForOutWhenUnconnected=off
  wires:
  NE_In/1 -> Assignment/1
  Data Store Read/1 -> Assignment/2
  Assignment/1 -> NE_IN_ForDigitalTacho/1  "NE_IN_ForDigitalTacho"

== system Mdl_Tacho/Mdl_Tacho_Task_sys/Subsystem/If Action Subsystem/Subsystem/Subsystem1 ==
  NE_IN_ForDigitalTacho_In : Inport
  Constant1 : Constant  Value=TACHO_COUNT_TWO
  Data Store Read2 : DataStoreRead  DataStoreName=DigtalTachoBuffIndex  IndexOptions=Index vector (dialog)  Indices=1  OutputSizes=1
  Data Store Write : DataStoreWrite  DataStoreName=DigitalTacho__Out  IndexOptions=Index vector (dialog)  Indices=1  OutputSizes=1
  If : If  NumInputs=2  IfExpression=u1 < u2
  If Action Subsystem : Subsystem  TreatAsAtomicUnit=on
  If Action Subsystem1 : Subsystem  TreatAsAtomicUnit=on
  Merge : Merge
  NE_IN_ForDigitalTacho_Out : Outport  VectorParamsAs1DForOutWhenUnconnected=off
  wires:
  Data Store Read2/1 -> If/1
  Constant1/1 -> If/2
  If/1 -> If Action Subsystem/Action
  If/2 -> If Action Subsystem1/Action
  NE_IN_ForDigitalTacho_In/1 -> If Action Subsystem1/1(NE_IN_ForDigitalTacho_In)
  Merge/1 -> Data Store Write/1, NE_IN_ForDigitalTacho_Out/1
  If Action Subsystem/1(Digital_Tacho_Out) -> Merge/1
  If Action Subsystem1/1(NE_IN_ForDigitalTacho__Out) -> Merge/2

== system Mdl_Tacho/Mdl_Tacho_Task_sys/Subsystem/NE1_Missing_Notify/If Action Subsystem/Debounce timer Subsystem ==
  Debounce_Count : Inport  OutDataTypeStr=uint8
  "ResetTimerStatus " : Inport  Port=2  OutDataTypeStr=boolean
  Constant1 : Constant  OutDataTypeStr=uint8  LockScale=on
  Constant2 : Constant  Value=TACHO_COUNT_INIT  OutDataTypeStr=uint8
  Constant7 : Constant  Value=0  OutDataTypeStr=boolean  LockScale=on
  DebounceIndex : UnitDelay  SampleTime=-1  StateName=DebounceIndex  HasFrameUpgradeWarning=on
  Display : Display
  Display1 : Display
  NE1_Status : Switch  Criteria=u2 ~= 0  OutDataTypeStr=uint8  RndMeth=Simplest  SaturateOnIntegerOverflow=off  InputSameDT=off
  Relational Operator1 : RelationalOperator  Operator=~=  OutDataTypeStr=boolean  InputSameDT=off
  Sum : Sum  OutDataTypeStr=uint8  RndMeth=Simplest
  Switch2 : Switch  Criteria=u2 ~= 0  OutDataTypeStr=uint8  RndMeth=Simplest  SaturateOnIntegerOverflow=off  InputSameDT=off
  check count : RelationalOperator  OutDataTypeStr=boolean  RndMeth=Simplest  InputSameDT=off
  TimerDebouncestatus : Outport  OutDataTypeStr=boolean  VectorParamsAs1DForOutWhenUnconnected=off
  wires:
  "ResetTimerStatus "/1 -> Relational Operator1/2
  Constant7/1 -> Relational Operator1/1
  Relational Operator1/1 -> Switch2/2
  Switch2/1 -> NE1_Status/3, check count/1  "current_count"
  Debounce_Count/1 -> check count/2, NE1_Status/1  "debounce_count"
  check count/1 -> Display1/1, TimerDebouncestatus/1, NE1_Status/2  "debounce_status"
  NE1_Status/1 -> Display/1, DebounceIndex/1
  Constant2/1 -> Switch2/1
  Sum/1 -> Switch2/3
  DebounceIndex/1 -> Sum/2
  Constant1/1 -> Sum/1

== system Mdl_Tacho/Mdl_Tacho_Task_sys/Subsystem/NE1_Missing_Notify/If Action Subsystem/Enabled Subsystem ==
  NE1_Value : Inport
  Enable : EnablePort
  Constant7 : Constant  Value=eEngineSpeedIn
  NE1_Recieve_Notify_Value : FunctionCaller  FunctionPrototype=NE1_Recieve_Notify_Value(NE1_SignalVal)  InputArgumentSpecifications=uint16(1)  OutputArgumentSpecifications=<Enter example>
  RxCan_SignalClearJustRcvdStatus1 : FunctionCaller  FunctionPrototype=RxCan_SignalClearJustRcvdStatus(SignalId)  InputArgumentSpecifications=tRxSignalId_type_instance(1)  OutputArgumentSpecifications=<Enter example>
  wires:
  Constant7/1 -> RxCan_SignalClearJustRcvdStatus1/1
  NE1_Value/1 -> NE1_Recieve_Notify_Value/1

== system Mdl_Tacho/Mdl_Tacho_Task_sys/Subsystem/If Action Subsystem/Average_Calculation/Subsystem/If Action Subsystem ==
  Action Port : ActionPort  ActionPortLabel=if(u1 ~= 0)
  Constant : Constant  Value=0  OutDataTypeStr=uint16
  "TachoCalculatedValue_Case1 " : Outport  VectorParamsAs1DForOutWhenUnconnected=off
  wires:
  Constant/1 -> "TachoCalculatedValue_Case1 "/1

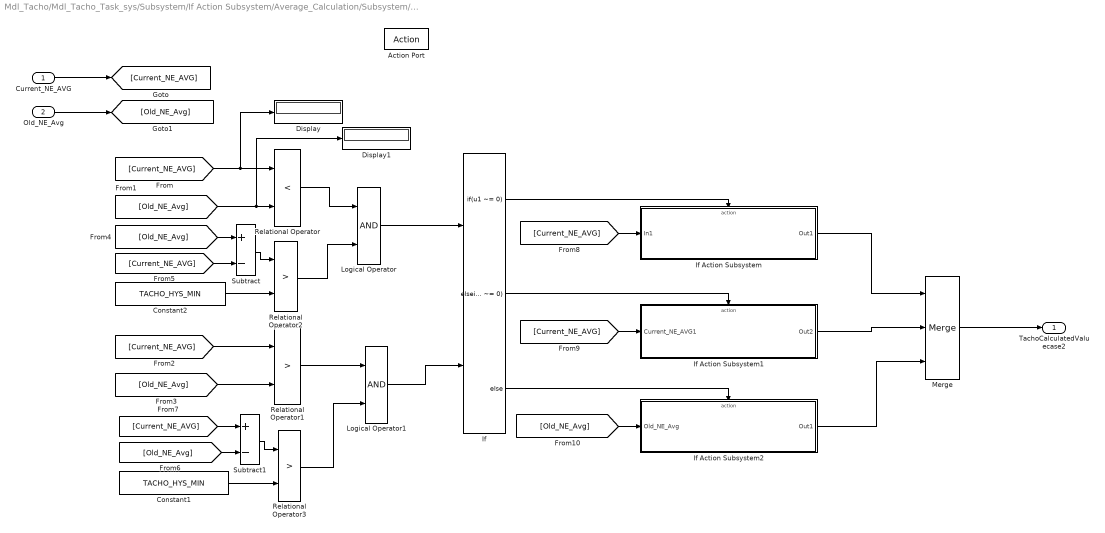
== system Mdl_Tacho/Mdl_Tacho_Task_sys/Subsystem/If Action Subsystem/Average_Calculation/Subsystem/If Action Subsystem1 ==
  Current_NE_AVG : Inport
  Old_NE_Avg : Inport  Port=2
  Action Port : ActionPort  ActionPortLabel=elseif(u2 ~= 0)
  Constant1 : Constant  Value=TACHO_HYS_MIN
  Constant2 : Constant  Value=TACHO_HYS_MIN
  Display : Display
  Display1 : Display
  If : If  NumInputs=2  IfExpression=u1 ~= 0  ElseIfExpressions=u2 ~= 0
  If Action Subsystem : Subsystem  TreatAsAtomicUnit=on
  If Action Subsystem1 : Subsystem  TreatAsAtomicUnit=on
  If Action Subsystem2 : Subsystem  TreatAsAtomicUnit=on
  Logical Operator : Logic  AllPortsSameDT=off  OutDataTypeStr=boolean
  Logical Operator1 : Logic  AllPortsSameDT=off  OutDataTypeStr=boolean
  Merge : Merge  Inputs=3
  Relational Operator : RelationalOperator  Operator=<  OutDataTypeStr=boolean  RndMeth=Simplest  InputSameDT=off
  Relational Operator1 : RelationalOperator  Operator=>  OutDataTypeStr=boolean  RndMeth=Simplest  InputSameDT=off
  Relational Operator2 : RelationalOperator  Operator=>  OutDataTypeStr=boolean  RndMeth=Simplest  InputSameDT=off
  Relational Operator3 : RelationalOperator  Operator=>  OutDataTypeStr=boolean  RndMeth=Simplest  InputSameDT=off
  Subtract : Sum  Inputs=+-  OutDataTypeStr=uint16  AccumDataTypeStr=uint16  RndMeth=Simplest
  Subtract1 : Sum  Inputs=+-  OutDataTypeStr=uint16  AccumDataTypeStr=uint16  RndMeth=Simplest
  TachoCalculatedValuecase2 : Outport  VectorParamsAs1DForOutWhenUnconnected=off
  wires:
  Current_NE_AVG/1 -> [Current_NE_AVG]
  Old_NE_Avg/1 -> [Old_NE_Avg]
  [Old_NE_Avg] -> Display1/1, Relational Operator/2
  [Current_NE_AVG] -> Display/1, Relational Operator/1
  [Current_NE_AVG] -> Relational Operator1/1
  [Old_NE_Avg] -> Relational Operator1/2
  If/1 -> If Action Subsystem/Action
  If/3 -> If Action Subsystem2/Action
  If/2 -> If Action Subsystem1/Action
  Relational Operator/1 -> Logical Operator/1
  [Old_NE_Avg] -> Subtract/1
  [Current_NE_AVG] -> Subtract/2
  Subtract/1 -> Relational Operator2/1
  Constant2/1 -> Relational Operator2/2
  Relational Operator2/1 -> Logical Operator/2
  Logical Operator/1 -> If/1
  Relational Operator3/1 -> Logical Operator1/2
  Constant1/1 -> Relational Operator3/2
  Subtract1/1 -> Relational Operator3/1
  [Current_NE_AVG] -> Subtract1/1
  [Old_NE_Avg] -> Subtract1/2
  Relational Operator1/1 -> Logical Operator1/1
  Logical Operator1/1 -> If/2
  [Current_NE_AVG] -> If Action Subsystem/1(In1)
  [Current_NE_AVG] -> If Action Subsystem1/1(Current_NE_AVG1)
  [Old_NE_Avg] -> If Action Subsystem2/1(Old_NE_Avg)
  Merge/1 -> TachoCalculatedValuecase2/1
  If Action Subsystem/1(Out1) -> Merge/1
  If Action Subsystem1/1(Out2) -> Merge/2
  If Action Subsystem2/1(Out1) -> Merge/3

== system Mdl_Tacho/Mdl_Tacho_Task_sys/Subsystem/If Action Subsystem/Average_Calculation/Subsystem/If Action Subsystem2 ==
  Current_NE_AVG : Inport
  Action Port : ActionPort  ActionPortLabel=else
  TachoCalculatedValuecase3 : Outport  VectorParamsAs1DForOutWhenUnconnected=off
  wires:
  Current_NE_AVG/1 -> TachoCalculatedValuecase3/1

== system Mdl_Tacho/Mdl_Tacho_Task_sys/Subsystem/If Action Subsystem/Enabled Subsystem/RPM Sampling/If Action Subsystem ==
  NE_AVE2 : Inport
  Action Port : ActionPort
  Constant1 : Constant  Value=true
  Constant2 : Constant  Value=TACHO_VAL_ONE_U16
  Data Store Read2 : DataStoreRead  DataStoreName=PeakUpValue  IndexOptions=Index vector (dialog)  Indices=1  OutputSizes=1
  Data Store Write : DataStoreWrite  DataStoreName=RevPeakOnOff  IndexOptions=Index vector (dialog)  Indices=1  OutputSizes=1
  Data Store Write1 : DataStoreWrite  DataStoreName=RevPeakValue  IndexOptions=Index vector (dialog)  Indices=1  OutputSizes=1
  Data Store Write2 : DataStoreWrite  DataStoreName=PeakDownValue  IndexOptions=Index vector (dialog)  Indices=1  OutputSizes=1
  Data Store Write3 : DataStoreWrite  DataStoreName=RevPeak_timer  IndexOptions=Index vector (dialog)  Indices=1  OutputSizes=1
  wires:
  Constant1/1 -> Data Store Write/1
  Data Store Read2/1 -> Data Store Write1/1
  NE_AVE2/1 -> Data Store Write2/1
  Constant2/1 -> Data Store Write3/1

== system Mdl_Tacho/Mdl_Tacho_Task_sys/Subsystem/If Action Subsystem/Enabled Subsystem/RPM Sampling/Subsystem ==
  NE_AVE2 : Inport
  Data Store Read1 : DataStoreRead  DataStoreName=PeakUpValue  IndexOptions=Index vector (dialog)  Indices=1  OutputSizes=1
  Data Store Write1 : DataStoreWrite  DataStoreName=PeakUpValue  IndexOptions=Index vector (dialog)  Indices=1  OutputSizes=1
  Equal : RelationalOperator  Operator=>  OutDataTypeStr=boolean  RndMeth=Simplest  InputSameDT=off
  Switch : Switch  Criteria=u2 ~= 0  SaturateOnIntegerOverflow=off  InputSameDT=off
  wires:
  Data Store Read1/1 -> Switch/3, Equal/2
  NE_AVE2/1 -> Switch/1, Equal/1
  Equal/1 -> Switch/2
  Switch/1 -> Data Store Write1/1

== system Mdl_Tacho/Mdl_Tacho_Task_sys/Subsystem/If Action Subsystem/Enabled Subsystem/RPM Sampling/Subsystem1 ==
  Constant1 : Constant  Value=TACHO_VAL_ZERO
  Data Store Read3 : DataStoreRead  DataStoreName=PeakDownValue  IndexOptions=Index vector (dialog)  Indices=1  OutputSizes=1
  Data Store Read4 : DataStoreRead  DataStoreName=PeakUpValue  IndexOptions=Index vector (dialog)  Indices=1  OutputSizes=1
  Data Store Read5 : DataStoreRead  DataStoreName=PeakUpValue  IndexOptions=Index vector (dialog)  Indices=1  OutputSizes=1
  Data Store Read6 : DataStoreRead  DataStoreName=PeakDownValue  IndexOptions=Index vector (dialog)  Indices=1  OutputSizes=1
  Equal1 : RelationalOperator  OutDataTypeStr=boolean  RndMeth=Simplest  InputSameDT=off
  Subtract1 : Sum  Inputs=+-
  Switch1 : Switch  Criteria=u2 ~= 0  SaturateOnIntegerOverflow=off  InputSameDT=off
  b : Outport  VectorParamsAs1DForOutWhenUnconnected=off
  wires:
  Data Store Read6/1 -> Equal1/2
  Data Store Read3/1 -> Subtract1/2
  Equal1/1 -> Switch1/2
  Constant1/1 -> Switch1/3
  Data Store Read5/1 -> Equal1/1
  Subtract1/1 -> Switch1/1
  Data Store Read4/1 -> Subtract1/1
  Switch1/1 -> b/1

== system Mdl_Tacho/Mdl_Tacho_Task_sys/Subsystem/If Action Subsystem/Enabled Subsystem/RPM Sampling/Subsystem2 ==
  NE_AVE2 : Inport
  Constant2 : Constant  Value=TACHO_VAL_ZERO
  Data Store Read1 : DataStoreRead  DataStoreName=PeakUpValue  IndexOptions=Index vector (dialog)  Indices=1  OutputSizes=1
  Data Store Read2 : DataStoreRead  DataStoreName=PeakUpValue  IndexOptions=Index vector (dialog)  Indices=1  OutputSizes=1
  Equal : RelationalOperator  OutDataTypeStr=boolean  RndMeth=Simplest  InputSameDT=off
  Subtract : Sum  Inputs=+-
  Switch : Switch  Criteria=u2 ~= 0  SaturateOnIntegerOverflow=off  InputSameDT=off
  a : Outport  VectorParamsAs1DForOutWhenUnconnected=off
  wires:
  Data Store Read1/1 -> Subtract/1
  Subtract/1 -> Switch/1
  Equal/1 -> Switch/2
  [NE_AVE2] -> Equal/2
  Data Store Read2/1 -> Equal/1
  Constant2/1 -> Switch/3
  NE_AVE2/1 -> [NE_AVE2]
  Switch/1 -> a/1
  [NE_AVE2] -> Subtract/2

== system Mdl_Tacho/Mdl_Tacho_Task_sys/Subsystem/If Action Subsystem/Enabled Subsystem/RPM Sampling/Timer ==
  Add : Sum
  Compare To Constant : simulink/Logic and Bit Operations/Compare To Constant  relop=<  const=TACHO_VAL_TWENTY  OutDataTypeStr=boolean
  Constant : Constant  Value=TACHO_COUNT_ONE
  Constant1 : Constant  Value=TACHO_VAL_ZERO
  Constant2 : Constant  Value=TACHO_VAL_ZERO
  Data Store Read : DataStoreRead  DataStoreName=PeakUpValue  IndexOptions=Index vector (dialog)  Indices=1  OutputSizes=1
  Data Store Read2 : DataStoreRead  DataStoreName=BufferIndex  IndexOptions=Index vector (dialog)  Indices=1  OutputSizes=1
  Data Store Read3 : DataStoreRead  DataStoreName=BufferIndex  IndexOptions=Index vector (dialog)  Indices=1  OutputSizes=1
  Data Store Write : DataStoreWrite  DataStoreName=BufferIndex  IndexOptions=Index vector (dialog)  Indices=1  OutputSizes=1
  Data Store Write1 : DataStoreWrite  DataStoreName=PeakUpValue  IndexOptions=Index vector (dialog)  Indices=1  OutputSizes=1
  Switch : Switch  Criteria=u2 ~= 0  Threshold=TACHO_VAL_TWENTY  SaturateOnIntegerOverflow=off  InputSameDT=off
  Switch1 : Switch  Criteria=u2 ~= 0  Threshold=TACHO_VAL_TWENTY  SaturateOnIntegerOverflow=off  InputSameDT=off
  wires:
  Data Store Read2/1 -> Compare To Constant/1
  Compare To Constant/1 -> Switch1/2, Switch/2
  Data Store Read3/1 -> Add/1
  Add/1 -> Switch/1
  Switch/1 -> Data Store Write/1
  Constant/1 -> Add/2
  Constant1/1 -> Switch/3
  Switch1/1 -> Data Store Write1/1
  Data Store Read/1 -> Switch1/1
  Constant2/1 -> Switch1/3

== system Mdl_Tacho/Mdl_Tacho_Task_sys/Subsystem/If Action Subsystem/Enabled Subsystem/Subsystem/If Action Subsystem ==
  NE_AVE2 : Inport
  Action Port : ActionPort
  Constant : Constant  Value=TACHO_VAL_ZERO
  Constant1 : Constant  Value=TACHO_VAL_ZERO_U16
  Data Store Write : DataStoreWrite  DataStoreName=PeakDownValue  IndexOptions=Index vector (dialog)  Indices=1  OutputSizes=1
  Data Store Write1 : DataStoreWrite  DataStoreName=PeakUpValue  IndexOptions=Index vector (dialog)  Indices=1  OutputSizes=1
  Data Store Write2 : DataStoreWrite  DataStoreName=BufferIndex  IndexOptions=Index vector (dialog)  Indices=1  OutputSizes=1
  wires:
  NE_AVE2/1 -> Data Store Write/1
  Constant/1 -> Data Store Write2/1
  Constant1/1 -> Data Store Write1/1

== system Mdl_Tacho/Mdl_Tacho_Task_sys/Subsystem/If Action Subsystem/Enabled Subsystem/Subsystem/If Action Subsystem1 ==
  Action Port : ActionPort
  Constant : Constant  Value=TACHO_VAL_ZERO
  Constant1 : Constant  Value=TACHO_VAL_ZERO_U16
  Data Store Write1 : DataStoreWrite  DataStoreName=PeakUpValue  IndexOptions=Index vector (dialog)  Indices=1  OutputSizes=1
  Data Store Write2 : DataStoreWrite  DataStoreName=BufferIndex  IndexOptions=Index vector (dialog)  Indices=1  OutputSizes=1
  wires:
  Constant1/1 -> Data Store Write1/1
  Constant/1 -> Data Store Write2/1
